simulink model "A2_2_Inverses_Pendel"  (R2023a)
settings: Solver=VariableStepAuto  StartTime=0.0  StopTime=10.0  RelTol=1e-3
values from neighbouring files (symbols this model uses):
  params = [ig c s ms CA CM]    [init_DSMS.m]    (also in init_DSMS_vorlage.m = [m c d g]; init_elast_Getriebe.m = [ig c s ms C_A_S C_M_S d]; init_inv.m = [m1 m2 l1 l2 s1 s2 C_1_S g d1 d2 m A_P B_P ig C_M]; init_inverse_pendel.m = [m1 m2 l1 l2 s1 s2 C_1_S g ig C_M_S])
  x1_ic = zeros(4,1)    [init_DSMS.m]    (also in init_DSMS_vorlage.m = zeros(2,1); init_elast_Getriebe.m; init_inv.m; init_inverse_pendel.m)
settings Model: Creator=Flo  LastModifiedBy=Flo

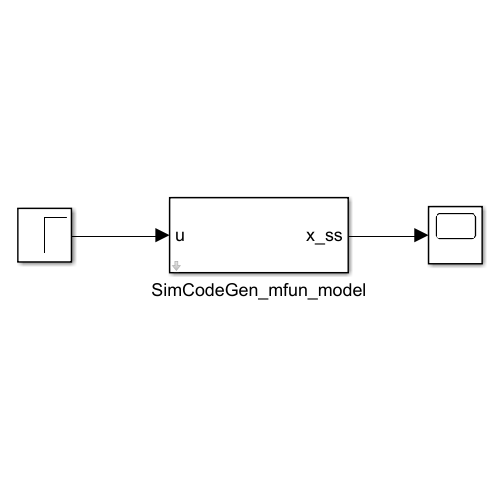
[thumbnail: Simulink's stored preview of the top-level diagram]
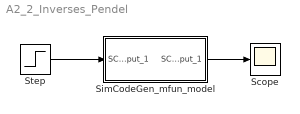
== system A2_2_Inverses_Pendel ==
  Scope : Scope
  SimCodeGen_mfun_model : Subsystem  mask{SC_param_0=params, SC_x1_ic=x1_ic}
      mask prompts: SC_param_0 "params"
      mask Display:
      | port_label('input', 1, 'u');
      | port_label('output', 1, 'x_ss');
  Step : Step  SampleTime=0
  wires:
  Step/1 -> SimCodeGen_mfun_model/1(SC_input_1)
  SimCodeGen_mfun_model/1(SC_output_1) -> Scope/1

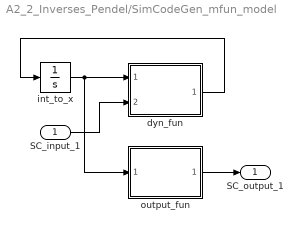
== system A2_2_Inverses_Pendel/SimCodeGen_mfun_model ==
  SC_input_1 : Inport
  dyn_fun : MATLAB Function  TreatAsAtomicUnit=on
  int_to_x : Integrator  InitialCondition=[SC_x1_ic]
  output_fun : MATLAB Function  TreatAsAtomicUnit=on
  SC_output_1 : Outport
  wires:
  int_to_x/1 -> dyn_fun/1(SC_state), output_fun/1(SC_state)
  SC_input_1/1 -> dyn_fun/2(SC_input_0)
  dyn_fun/1(SC_state_dot) -> int_to_x/1
  output_fun/1(SC_output_0) -> SC_output_1/1

== matlab function A2_2_Inverses_Pendel/SimCodeGen_mfun_model/dyn_fun ==
  data: SC_state input size=[4]; SC_state_dot output size=[4]; SC_input_0 input size=[1]; SC_param_0 parameter
function SC_state_dot  = dyn_fun(SC_state, SC_input_0, SC_param_0)
    SC_state_dot = zeros(4, 1);
    SC_state_x_0 = SC_state(1:4);
    SC_eval = zeros(4,1);
    SC_eval(1) = SC_state_x_0(3);
    SC_eval(2) = SC_state_x_0(4);
    t1 = SC_state_x_0(2);
    t2 = cos(t1);
    t3 = t2 ^ 2;
    t4 = SC_param_0(3);
    t6 = SC_param_0(2);
    t5 = SC_eval(1);
    t7 = t5 ^ 2;
    t9 = SC_param_0(6);
    t12 = (t9 ^ 2);
    t16 = SC_param_0(8);
    t17 = (t4 * t16);
    t8 = SC_eval(2);
    t23 = t8 ^ 2;
    t27 = sin(t1);
    t31 = SC_input_0(1) * SC_param_0(9);
    t33 = (t4 ^ 2);
    t36 = t27 ^ 2;
    t40 = SC_param_0(5) ^ 2;
    t41 = t40 * SC_param_0(1);
    t42 = SC_param_0(7);
    t24 = t4 * t6;
    SC_eval(3) = ((t3 * t24 * t9 * t7 + ((-2 * t12 * t5 * t8 + t17) * t6 + t17) * t2 - t24 * t9 * t23) * t27 + t31) / (t36 * (t33 + t12) * t6 + t41 + t42);
    t47 = t36 * t12 * t6;
    t50 = t6 * t33;
    SC_eval(4) = 0.1e1 / t9 / (-t3 * t33 * t6 + t41 + t42 + t47 + t50) * (-t2 * t4 * (t6 * t9 * t8 * (0.2e1 * t2 * t5 * t9 + (t4 * t8)) * t27 - t31) - (-(t2 * t7 * t9 + t16) * t6 - t16) * t27 / t6 * (t47 + t50 + t41 + t42));
    SC_state_dot(1:4) = SC_eval(1:4);
end

== matlab function A2_2_Inverses_Pendel/SimCodeGen_mfun_model/output_fun ==
  data: SC_state input size=[4]; SC_output_0 output size=[4]; SC_param_0 parameter size=[9]
function SC_output_0  = y_fun(SC_state, SC_param_0)
    SC_output_0 = zeros(4,1);
    SC_state_x_0 = SC_state(1:4);
    SC_output_0(1) = SC_state_x_0(1);
    SC_output_0(2) = SC_state_x_0(2);
    SC_output_0(3) = SC_state_x_0(3);
    SC_output_0(4) = SC_state_x_0(4);
end
